simulink model "MDR_AA_TMD_Intercepteur"  (R2019b)
settings: Solver=ode4  StartTime=0.0  StopTime=Inf  FixedStep=0.01  RelTol=1e-3
values from neighbouring files (symbols this model uses):
  stdatm = [0 100 200 300 400 500 600 700 800 900 1000 1100 ... (4305 elements, 861x5)]    [stdatm.mat]
undefined symbols (not defined in the file or in its folder): Aero_Struct_CM, Aero_TMD, e0_0, e1_0, e2_0, e3_0, magnitude, Masse_Inertie_TMD, pow, Propu_TMD, Simu_TMD, Vm_0, xme_0
libraries: simulink x17
(part 3 of 4)

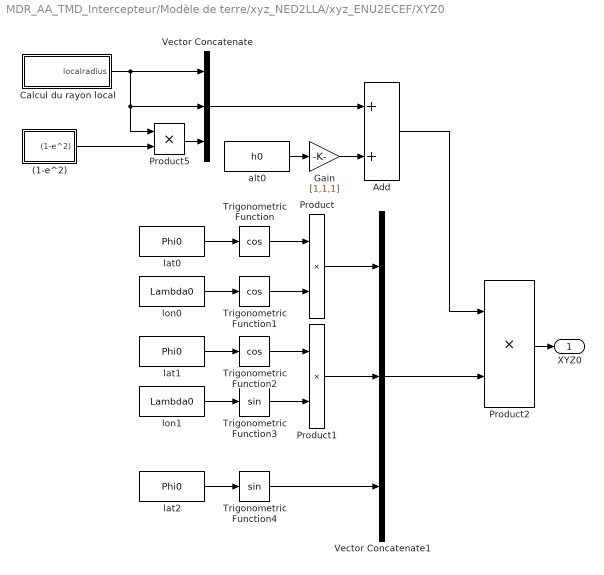
== system MDR_AA_TMD_Intercepteur/Modèle de terre/xyz_NED2LLA/xyz_ENU2ECEF/XYZ0 ==
  (1-e^2) : Subsystem
  Add : Sum
  Calcul du rayon local : Subsystem
  Gain : Gain  Gain=[1,1,1]
  Product{,1..2,5} (4 alike) : Product
  Trigonometric Function : Trigonometry  Operator=cos
  Trigonometric Function1 : Trigonometry  Operator=cos
  Trigonometric Function2 : Trigonometry  Operator=cos
  Trigonometric Function3 : Trigonometry
  Trigonometric Function4 : Trigonometry
  Vector Concatenate : Concatenate  NumInputs=3
  Vector Concatenate1 : Concatenate  NumInputs=3
  alt0 : Constant  Value=h0
  lat0 : Constant  Value=Phi0
  lat1 : Constant  Value=Phi0
  lat2 : Constant  Value=Phi0
  lon0 : Constant  Value=Lambda0
  lon1 : Constant  Value=Lambda0
  XYZ0 : Outport  VectorParamsAs1DForOutWhenUnconnected=off
  wires:
  Calcul du rayon local/1(localradius) -> Product5/1, Vector Concatenate/2, Vector Concatenate/1
  Product2/1 -> XYZ0/1
  Trigonometric Function4/1 -> Vector Concatenate1/3
  Add/1 -> Product2/1
  Product5/1 -> Vector Concatenate/3
  lon1/1 -> Trigonometric Function3/1
  Trigonometric Function2/1 -> Product1/1
  Trigonometric Function3/1 -> Product1/2
  Trigonometric Function1/1 -> Product/2
  Product1/1 -> Vector Concatenate1/2
  Gain/1 -> Add/2
  Trigonometric Function/1 -> Product/1
  lat1/1 -> Trigonometric Function2/1
  Product/1 -> Vector Concatenate1/1
  alt0/1 -> Gain/1
  lon0/1 -> Trigonometric Function1/1
  lat0/1 -> Trigonometric Function/1
  Vector Concatenate/1 -> Add/1
  (1-e^2)/1((1-e^2)) -> Product5/2
  lat2/1 -> Trigonometric Function4/1
  Vector Concatenate1/1 -> Product2/2

== system MDR_AA_TMD_Intercepteur/Cible/Cible Cinématique v1.1/Actionneur Simulight/Retard Angle/Gestion division par 0 ==
  Zero_Possible : Inport
  IC : InitialCondition  Value=0.01
  Memory : Memory
  Switch : Switch  Criteria=u2 ~= 0
  Non_zero : Outport  VectorParamsAs1DForOutWhenUnconnected=off
  wires:
  IC/1 -> Non_zero/1
  Memory/1 -> Switch/3
  Switch/1 -> IC/1, Memory/1
  Zero_Possible/1 -> Switch/2, Switch/1

== system MDR_AA_TMD_Intercepteur/Cible/Cible Cinématique v1.1/Actionneur Simulight1/Retard Angle/Gestion division par 0 ==
  Zero_Possible : Inport
  IC : InitialCondition  Value=0.01
  Memory : Memory
  Switch : Switch  Criteria=u2 ~= 0
  Non_zero : Outport  VectorParamsAs1DForOutWhenUnconnected=off
  wires:
  IC/1 -> Non_zero/1
  Memory/1 -> Switch/3
  Switch/1 -> IC/1, Memory/1
  Zero_Possible/1 -> Switch/2, Switch/1

== system MDR_AA_TMD_Intercepteur/Cible/Cible Cinématique v1.1/Cinématique 6ddl Simulight avec pilotage en force/Calcul de la vitesse engin dans le repère inertiel/Quaternion2DCM ==
  note: Output
  note: Assemble Body-Inertial DCM
  Quaternion : Inport  PortDimensions=[4 1]
  1-2q1^2-2q2^2 : Fcn  Expr=1-2*u(2)^2-2*u(3)^2
  1-2q1^2-2q3^2 : Fcn  Expr=1-2*u(2)^2-2*u(4)^2
  1-2q2^2-2q3^2 : Fcn  Expr=1-2*u(3)^2-2*u(4)^2
  2q1q2+2q0q3 : Fcn  Expr=2*u(2)*u(3)+2*u(1)*u(4)
  2q1q2-2q0q3 : Fcn  Expr=2*u(2)*u(3)-2*u(1)*u(4)
  2q1q3+2q0q2 : Fcn  Expr=2*u(2)*u(4)+2*u(1)*u(3)
  2q1q3-2q0q2 : Fcn  Expr=2*u(2)*u(4)-2*u(1)*u(3)
  2q2q3+2q0q1 : Fcn  Expr=2*u(3)*u(4)+2*u(1)*u(2)
  2q2q3-2q0q1 : Fcn  Expr=2*u(3)*u(4)-2*u(1)*u(2)
  Math Function : Math  Operator=transpose  SaturateOnIntegerOverflow=on
  Rbi Matrix : Concatenate  NumInputs=3  Mode=Multidimensional array  ConcatenateDimension=2
  Rbi Col1 : Concatenate  NumInputs=3  Mode=Multidimensional array
  Rbi Col2 : Concatenate  NumInputs=3  Mode=Multidimensional array
  Rbi Col3 : Concatenate  NumInputs=3  Mode=Multidimensional array
  DCM : Outport  VectorParamsAs1DForOutWhenUnconnected=off
  wires:
  Math Function/1 -> DCM/1
  Rbi Matrix/1 -> Math Function/1
  Rbi Col1/1 -> Rbi Matrix/1
  1-2q2^2-2q3^2/1 -> Rbi Col1/1
  2q1q2+2q0q3/1 -> Rbi Col1/2
  2q1q3-2q0q2/1 -> Rbi Col1/3
  2q1q2-2q0q3/1 -> Rbi Col2/1
  1-2q1^2-2q3^2/1 -> Rbi Col2/2
  2q2q3+2q0q1/1 -> Rbi Col2/3
  2q1q3+2q0q2/1 -> Rbi Col3/1
  2q2q3-2q0q1/1 -> Rbi Col3/2
  1-2q1^2-2q2^2/1 -> Rbi Col3/3
  Rbi Col2/1 -> Rbi Matrix/2
  Rbi Col3/1 -> Rbi Matrix/3
  Quaternion/1 -> 1-2q2^2-2q3^2/1, 2q1q2+2q0q3/1, 2q1q3-2q0q2/1, 2q1q2-2q0q3/1, 2q2q3-2q0q1/1, 1-2q1^2-2q2^2/1, 2q1q3+2q0q2/1, 2q2q3+2q0q1/1, 1-2q1^2-2q3^2/1

== system MDR_AA_TMD_Intercepteur/Cible/Cible Cinématique v1.1/Cinématique 6ddl Simulight avec pilotage en force/Calcul des pqr/pqr_a ==
  AlphaR : Inport
  BetaR : Inport  Port=2
  Constant : Constant  Value=0
  Vector Concatenate : Concatenate  NumInputs=3
  dérive alpha/beta : Subsystem
  pqr_a : Outport  VectorParamsAs1DForOutWhenUnconnected=off
  wires:
  AlphaR/1 -> dérive alpha/beta/1(AlphaR)
  BetaR/1 -> dérive alpha/beta/2(BetaR)
  dérive alpha/beta/2(dBetaR) -> Vector Concatenate/3
  dérive alpha/beta/1(dAlphaR) -> Vector Concatenate/2
  Constant/1 -> Vector Concatenate/1
  Vector Concatenate/1 -> pqr_a/1

== system MDR_AA_TMD_Intercepteur/Cible/Cible Cinématique v1.1/Cinématique 6ddl Simulight avec pilotage en force/Calcul des pqr/pqr_b ==
  Ab : Inport
  Vb : Inport  Port=2
  Divide : Product  Inputs=*/
  Gain : Gain  Gain=[0 -1 1]
  Selector : Selector  InputPortWidth=3  IndexOptions=Index vector (dialog)  Indices=[1]  OutputSizes=1
  Selector1 : Selector  InputPortWidth=3  IndexOptions=Index vector (dialog)  Indices=[1 3 2]  OutputSizes=1
  pqr_b : Outport  VectorParamsAs1DForOutWhenUnconnected=off
  wires:
  Selector/1 -> Divide/2
  Ab/1 -> Selector1/1
  Vb/1 -> Selector/1
  Divide/1 -> Gain/1
  Gain/1 -> pqr_b/1
  Selector1/1 -> Divide/1

== system MDR_AA_TMD_Intercepteur/Cible/Cible Cinématique v1.1/Cinématique 6ddl Simulight avec pilotage en force/Equations des forces/Gestion de sortie de rampe ==
  Fm : Inport
  Compare To Constant : simulink/Logic and Bit Operations/Compare To Constant  relop=>  const=Longueur_Missile/1000  OutDataTypeStr=boolean
  Integrator : Integrator
  Integrator1 : Integrator  InitialCondition=[0 0 0]
  Norme : Subsystem  mask(Norme){}
      mask help: Calcul la norme quadratique d'un vecteur.
      mask Help: eval('OpenHelp(''A3_NG.mdl'', ''Help\html\A3_NG_Model_Norme.html'')');
  Saturation : Saturate  UpperLimit=inf  LowerLimit=0
  Selector1 : Selector  InputPortWidth=3  IndexOptions=Index vector (dialog)  Indices=[1]  OutputSizes=1
  Sortie_Rampe : Outport  VectorParamsAs1DForOutWhenUnconnected=off
  wires:
  Integrator1/1 -> Norme/1(V)
  Norme/1(||V||) -> Compare To Constant/1
  Integrator/1 -> Integrator1/1
  Compare To Constant/1 -> Sortie_Rampe/1
  Selector1/1 -> Saturation/1
  Saturation/1 -> Integrator/1
  Fm/1 -> Selector1/1

== system MDR_AA_TMD_Intercepteur/Cible/Cible Cinématique v1.1/Cinématique 6ddl Simulight avec pilotage en force/Equations des forces/Sous contrainte de la rampe, effort uniquement sur l'axe longitudinal ==
  F : Inport
  Constant : Constant  Value=0
  Constant1 : Constant  Value=0
  Saturation : Saturate  UpperLimit=inf  LowerLimit=0
  Selector1 : Selector  InputPortWidth=3  IndexOptions=Index vector (dialog)  Indices=[1]  OutputSizes=1
  Vector Concatenate : Concatenate  NumInputs=3
  Fx : Outport  VectorParamsAs1DForOutWhenUnconnected=off
  wires:
  F/1 -> Selector1/1
  Selector1/1 -> Saturation/1
  Saturation/1 -> Vector Concatenate/1
  Vector Concatenate/1 -> Fx/1
  Constant/1 -> Vector Concatenate/2
  Constant1/1 -> Vector Concatenate/3

== system MDR_AA_TMD_Intercepteur/Cible/Cible Cinématique v1.1/Cinématique 6ddl Simulight avec pilotage en force/Equations des forces/U^V ==
  a(1) a(2) a(3) : Inport
  b(1) b(2) b(3) : Inport  Port=2
  Product : Product  SaturateOnIntegerOverflow=on  RndMeth=Zero  InputSameDT=on  OutDataTypeStr=Inherit: Same as first input
  Product1 : Product  SaturateOnIntegerOverflow=on  RndMeth=Zero  InputSameDT=on  OutDataTypeStr=Inherit: Same as first input
  Selector : Selector  InputPortWidth=3  IndexOptions=Index vector (dialog)  Indices=[2 3 1]  OutputSizes=1
  Selector1 : Selector  InputPortWidth=3  IndexOptions=Index vector (dialog)  Indices=[3 1 2]  OutputSizes=1
  Selector2 : Selector  InputPortWidth=3  IndexOptions=Index vector (dialog)  Indices=[2 3 1]  OutputSizes=1
  Selector3 : Selector  InputPortWidth=3  IndexOptions=Index vector (dialog)  Indices=[3 1 2]  OutputSizes=1
  Sum : Sum  Inputs=+|-  SaturateOnIntegerOverflow=on  InputSameDT=on  OutDataTypeStr=Inherit: Same as first input
  c(1) c(2) c(3) : Outport  VectorParamsAs1DForOutWhenUnconnected=off
  wires:
  Sum/1 -> c(1) c(2) c(3)/1
  b(1) b(2) b(3)/1 -> Selector1/1, Selector2/1
  Selector/1 -> Product/1
  a(1) a(2) a(3)/1 -> Selector/1, Selector3/1
  Product/1 -> Sum/1
  Selector1/1 -> Product/2
  Product1/1 -> Sum/2
  Selector2/1 -> Product1/2
  Selector3/1 -> Product1/1

== system MDR_AA_TMD_Intercepteur/Cible/Cible Cinématique v1.1/Cinématique 6ddl Simulight avec pilotage en force/Pesanteur/Inert2Miss ==
  Euler : Inport
  U : Inport  Port=2
  Euler2DCM : Subsystem  mask(Euler2DCM){}
      mask help:
      | Calcul la matrice de passage DCM (Direct Cosine Matrix) à partir des angles d'Euler.
      |
      | DCM :=[
      | [c(theta)c(psi)	-c(phi)s(psi)+s(phi)s(theta)c(psi)	s(phi)s(psi)+c(phi)s(theta)c(psi)
      |
      | c(theta)s(psi)	c(phi)c(psi)+s(phi)s(theta)s(psi)	-s(phi)c(psi)+c(phi)s(theta)s(psi)
      |
      | -s(theta)		s(phi)c(theta)			c(phi)c(theta)
      | ]^T
      | où c correspond à cos,  et s correspond à sin
      mask Help: eval('OpenHelp(''A3_NG.mdl'', ''Help\html\A3_NG_Model_Euler2DCM.html'')');
  Product : Product  Multiplication=Matrix(*)  RndMeth=Zero
  V : Outport  VectorParamsAs1DForOutWhenUnconnected=off
  wires:
  Euler2DCM/1(DCM) -> Product/1
  Product/1 -> V/1
  U/1 -> Product/2
  Euler/1 -> Euler2DCM/1(Euler)

== system MDR_AA_TMD_Intercepteur/Cible/Cible Cinématique v1.1/Cinématique 6ddl Simulight avec pilotage en force/pqr2Quaternion/Euler2Quaternion ==
  note: Sources
  note: Attitude trigonometry
  Euler : Inport  PortDimensions=[3 1]
  1/2 : Gain  Gain=1/2  SaturateOnIntegerOverflow=on  OutDataTypeStr=Inherit: Same as input  ParamDataTypeStr=Inherit: Same as input
  Demux : Demux  Outputs=3
  Fcn4 : Fcn  Expr=u(2)*u(4)*u(6)+u(1)*u(3)*u(5)
  Fcn5 : Fcn  Expr=u(1)*u(4)*u(6)-u(2)*u(3)*u(5)
  Fcn6 : Fcn  Expr=u(2)*u(3)*u(6)+u(1)*u(4)*u(5)
  Fcn7 : Fcn  Expr=u(2)*u(4)*u(5)-u(1)*u(3)*u(6)
  Mux1 : Mux  Inputs=6
  Mux3 : Mux
  cos(phi/2) : Trigonometry  Operator=cos
  cos(psi/2) : Trigonometry  Operator=cos
  cos(theta/2) : Trigonometry  Operator=cos
  sin(phi/2) : Trigonometry
  sin(psi/2) : Trigonometry
  sin(theta/2) : Trigonometry
  Quaternion : Outport  VectorParamsAs1DForOutWhenUnconnected=off
  wires:
  Fcn7/1 -> Mux3/4
  Fcn6/1 -> Mux3/3
  Fcn5/1 -> Mux3/2
  Fcn4/1 -> Mux3/1
  Mux3/1 -> Quaternion/1
  Mux1/1 -> Fcn7/1, Fcn6/1, Fcn4/1, Fcn5/1
  cos(psi/2)/1 -> Mux1/6
  sin(psi/2)/1 -> Mux1/5
  cos(theta/2)/1 -> Mux1/4
  sin(theta/2)/1 -> Mux1/3
  cos(phi/2)/1 -> Mux1/2
  sin(phi/2)/1 -> Mux1/1
  Euler/1 -> 1/2/1
  1/2/1 -> Demux/1
  Demux/1 -> sin(phi/2)/1, cos(phi/2)/1
  Demux/2 -> cos(theta/2)/1, sin(theta/2)/1
  Demux/3 -> cos(psi/2)/1, sin(psi/2)/1

== system MDR_AA_TMD_Intercepteur/Cible/Cible Cinématique v1.1/Cinématique 6ddl Simulight avec pilotage en force/pqr2Quaternion/Norme ==
  V : Inport
  Dot Product : DotProduct  InputSameDT=on  OutDataTypeStr=Inherit: Inherit via internal rule
  Sqrt : Math  Operator=sqrt  SaturateOnIntegerOverflow=on
  ||V|| : Outport  VectorParamsAs1DForOutWhenUnconnected=off
  wires:
  Sqrt/1 -> ||V||/1
  V/1 -> Dot Product/2, Dot Product/1
  Dot Product/1 -> Sqrt/1

== system MDR_AA_TMD_Intercepteur/Cible/Cible Cinématique v1.1/Cinématique 6ddl Simulight avec pilotage en force/pqr2Quaternion/pqr to eidot ==
  pqr : Inport
  e0e1e2e3 : Inport  Port=2
  Gain : Gain  Gain=100  SaturateOnIntegerOverflow=on  OutDataTypeStr=Inherit: Same as input  ParamDataTypeStr=Inherit: Same as input
  Mux1 : Mux  Inputs=[3 4 1]
  Mux2 : Mux
  e0dot : Fcn  Expr=-0.5 * ( u[5]*u[1]+u[6]*u[2]+u[7]*u[3] )
  e1dot : Fcn  Expr=0.5 * ( u[4]*u[1]+u[6]*u[3]-u[7]*u[2] )
  e2dot : Fcn  Expr=0.5 * ( u[4]*u[2]+u[7]*u[1]-u[5]*u[3] )
  e3dot : Fcn  Expr=0.5 * ( u[4]*u[3]+u[5]*u[2]-u[6]*u[1] )
  lambda : Fcn  Expr=1-( pow(u[1],2) + pow(u[2],2) + pow(u[3],2) + pow(u[4],2) )
  eidot : Outport  VectorParamsAs1DForOutWhenUnconnected=off
  wires:
  e0e1e2e3/1 -> Mux1/2, lambda/1
  Gain/1 -> Mux1/3
  lambda/1 -> Gain/1
  e3dot/1 -> Mux2/4
  Mux1/1 -> e3dot/1, e2dot/1, e1dot/1, e0dot/1
  e2dot/1 -> Mux2/3
  e1dot/1 -> Mux2/2
  e0dot/1 -> Mux2/1
  pqr/1 -> Mux1/1
  Mux2/1 -> eidot/1

== system MDR_AA_TMD_Intercepteur/Cible/Cible Cinématique v1.1/Pilote 2 axes Simulight à partir de gradient/Alpha commandé - Plan de tangage/Zero Offset ==
  In : Inport
  Abs : Abs  SaturateOnIntegerOverflow=on
  Constant : Constant  Value=tol
  Non-zero Sign : Subsystem  mask(Non-zero sign){}
      mask help: Sign function outputs 1 for input greater than or equal to 0, and -1 otherwise.
  Product : Product  SaturateOnIntegerOverflow=on  RndMeth=Zero  InputSameDT=on  OutDataTypeStr=Inherit: Same as first input
  Switch : Switch  Threshold=tol  SaturateOnIntegerOverflow=on  InputSameDT=on
  Out : Outport  VectorParamsAs1DForOutWhenUnconnected=off
  wires:
  Switch/1 -> Out/1
  Product/1 -> Switch/3
  Constant/1 -> Product/2
  Non-zero Sign/1(Out) -> Product/1
  Abs/1 -> Switch/2
  In/1 -> Abs/1, Non-zero Sign/1(In), Switch/1

== system MDR_AA_TMD_Intercepteur/Cible/Cible Cinématique v1.1/Pilote 2 axes Simulight à partir de gradient/Beta commandé - Plan de lacet/Zero Offset ==
  In : Inport
  Abs : Abs  SaturateOnIntegerOverflow=on
  Constant : Constant  Value=tol
  Non-zero Sign : Subsystem  mask(Non-zero sign){}
      mask help: Sign function outputs 1 for input greater than or equal to 0, and -1 otherwise.
  Product : Product  SaturateOnIntegerOverflow=on  RndMeth=Zero  InputSameDT=on  OutDataTypeStr=Inherit: Same as first input
  Switch : Switch  Threshold=tol  SaturateOnIntegerOverflow=on  InputSameDT=on
  Out : Outport  VectorParamsAs1DForOutWhenUnconnected=off
  wires:
  In/1 -> Switch/1, Non-zero Sign/1(In), Abs/1
  Abs/1 -> Switch/2
  Non-zero Sign/1(Out) -> Product/1
  Constant/1 -> Product/2
  Product/1 -> Switch/3
  Switch/1 -> Out/1

== system MDR_AA_TMD_Intercepteur/Intercepteur_TMD/Auto-Directeur/Autodirecteur Parfait v1.0/Calcul du vecteur rotation instantané de la droite missile//but dans le repère inertiel/Norme ==
  V : Inport
  Dot Product : DotProduct  InputSameDT=on  OutDataTypeStr=Inherit: Inherit via internal rule
  Sqrt : Math  Operator=sqrt  SaturateOnIntegerOverflow=on
  ||V|| : Outport  VectorParamsAs1DForOutWhenUnconnected=off
  wires:
  Sqrt/1 -> ||V||/1
  V/1 -> Dot Product/2, Dot Product/1
  Dot Product/1 -> Sqrt/1

== system MDR_AA_TMD_Intercepteur/Intercepteur_TMD/Auto-Directeur/Autodirecteur Parfait v1.0/Calcul du vecteur rotation instantané de la droite missile//but dans le repère inertiel/U^V ==
  a(1) a(2) a(3) : Inport
  b(1) b(2) b(3) : Inport  Port=2
  Product : Product  SaturateOnIntegerOverflow=on  RndMeth=Zero  InputSameDT=on  OutDataTypeStr=Inherit: Same as first input
  Product1 : Product  SaturateOnIntegerOverflow=on  RndMeth=Zero  InputSameDT=on  OutDataTypeStr=Inherit: Same as first input
  Selector : Selector  InputPortWidth=3  IndexOptions=Index vector (dialog)  Indices=[2 3 1]  OutputSizes=1
  Selector1 : Selector  InputPortWidth=3  IndexOptions=Index vector (dialog)  Indices=[3 1 2]  OutputSizes=1
  Selector2 : Selector  InputPortWidth=3  IndexOptions=Index vector (dialog)  Indices=[2 3 1]  OutputSizes=1
  Selector3 : Selector  InputPortWidth=3  IndexOptions=Index vector (dialog)  Indices=[3 1 2]  OutputSizes=1
  Sum : Sum  Inputs=+|-  SaturateOnIntegerOverflow=on  InputSameDT=on  OutDataTypeStr=Inherit: Same as first input
  c(1) c(2) c(3) : Outport  VectorParamsAs1DForOutWhenUnconnected=off
  wires:
  Sum/1 -> c(1) c(2) c(3)/1
  b(1) b(2) b(3)/1 -> Selector1/1, Selector2/1
  Selector/1 -> Product/1
  a(1) a(2) a(3)/1 -> Selector/1, Selector3/1
  Product/1 -> Sum/1
  Selector1/1 -> Product/2
  Product1/1 -> Sum/2
  Selector2/1 -> Product1/2
  Selector3/1 -> Product1/1

== system MDR_AA_TMD_Intercepteur/Intercepteur_TMD/Auto-Directeur/Autodirecteur Parfait v1.0/Changement de repère inertiel -> miss/Inert2Miss1 ==
  Euler : Inport
  U : Inport  Port=2
  Euler2DCM : Subsystem  mask(Euler2DCM){}
      mask help:
      | Calcul la matrice de passage DCM (Direct Cosine Matrix) à partir des angles d'Euler.
      |
      | DCM :=[
      | [c(theta)c(psi)	-c(phi)s(psi)+s(phi)s(theta)c(psi)	s(phi)s(psi)+c(phi)s(theta)c(psi)
      |
      | c(theta)s(psi)	c(phi)c(psi)+s(phi)s(theta)s(psi)	-s(phi)c(psi)+c(phi)s(theta)s(psi)
      |
      | -s(theta)		s(phi)c(theta)			c(phi)c(theta)
      | ]^T
      | où c correspond à cos,  et s correspond à sin
      mask Help: eval('OpenHelp(''A3_NG.mdl'', ''Help\html\A3_NG_Model_Euler2DCM.html'')');
  Product : Product  Multiplication=Matrix(*)  RndMeth=Zero
  V : Outport  VectorParamsAs1DForOutWhenUnconnected=off
  wires:
  Euler2DCM/1(DCM) -> Product/1
  Product/1 -> V/1
  U/1 -> Product/2
  Euler/1 -> Euler2DCM/1(Euler)

== system MDR_AA_TMD_Intercepteur/Intercepteur_TMD/Auto-Directeur/Autodirecteur Parfait v1.0/Site et Gisement de la droite missile//but dans le repère inertiel/Norme ==
  V : Inport
  Dot Product : DotProduct  InputSameDT=on  OutDataTypeStr=Inherit: Inherit via internal rule
  Sqrt : Math  Operator=sqrt  SaturateOnIntegerOverflow=on
  ||V|| : Outport  VectorParamsAs1DForOutWhenUnconnected=off
  wires:
  Sqrt/1 -> ||V||/1
  V/1 -> Dot Product/2, Dot Product/1
  Dot Product/1 -> Sqrt/1

== system MDR_AA_TMD_Intercepteur/Intercepteur_TMD/Bloc Cinématique/Cinématique 6ddl Simulight avec pilotage en force/Calcul de la vitesse engin dans le repère inertiel/Quaternion2DCM ==
  note: Output
  note: Assemble Body-Inertial DCM
  Quaternion : Inport  PortDimensions=[4 1]
  1-2q1^2-2q2^2 : Fcn  Expr=1-2*u(2)^2-2*u(3)^2
  1-2q1^2-2q3^2 : Fcn  Expr=1-2*u(2)^2-2*u(4)^2
  1-2q2^2-2q3^2 : Fcn  Expr=1-2*u(3)^2-2*u(4)^2
  2q1q2+2q0q3 : Fcn  Expr=2*u(2)*u(3)+2*u(1)*u(4)
  2q1q2-2q0q3 : Fcn  Expr=2*u(2)*u(3)-2*u(1)*u(4)
  2q1q3+2q0q2 : Fcn  Expr=2*u(2)*u(4)+2*u(1)*u(3)
  2q1q3-2q0q2 : Fcn  Expr=2*u(2)*u(4)-2*u(1)*u(3)
  2q2q3+2q0q1 : Fcn  Expr=2*u(3)*u(4)+2*u(1)*u(2)
  2q2q3-2q0q1 : Fcn  Expr=2*u(3)*u(4)-2*u(1)*u(2)
  Math Function : Math  Operator=transpose  SaturateOnIntegerOverflow=on
  Rbi Matrix : Concatenate  NumInputs=3  Mode=Multidimensional array  ConcatenateDimension=2
  Rbi Col1 : Concatenate  NumInputs=3  Mode=Multidimensional array
  Rbi Col2 : Concatenate  NumInputs=3  Mode=Multidimensional array
  Rbi Col3 : Concatenate  NumInputs=3  Mode=Multidimensional array
  DCM : Outport  VectorParamsAs1DForOutWhenUnconnected=off
  wires:
  Math Function/1 -> DCM/1
  Rbi Matrix/1 -> Math Function/1
  Rbi Col1/1 -> Rbi Matrix/1
  1-2q2^2-2q3^2/1 -> Rbi Col1/1
  2q1q2+2q0q3/1 -> Rbi Col1/2
  2q1q3-2q0q2/1 -> Rbi Col1/3
  2q1q2-2q0q3/1 -> Rbi Col2/1
  1-2q1^2-2q3^2/1 -> Rbi Col2/2
  2q2q3+2q0q1/1 -> Rbi Col2/3
  2q1q3+2q0q2/1 -> Rbi Col3/1
  2q2q3-2q0q1/1 -> Rbi Col3/2
  1-2q1^2-2q2^2/1 -> Rbi Col3/3
  Rbi Col2/1 -> Rbi Matrix/2
  Rbi Col3/1 -> Rbi Matrix/3
  Quaternion/1 -> 1-2q2^2-2q3^2/1, 2q1q2+2q0q3/1, 2q1q3-2q0q2/1, 2q1q2-2q0q3/1, 2q2q3-2q0q1/1, 1-2q1^2-2q2^2/1, 2q1q3+2q0q2/1, 2q2q3+2q0q1/1, 1-2q1^2-2q3^2/1

== system MDR_AA_TMD_Intercepteur/Intercepteur_TMD/Bloc Cinématique/Cinématique 6ddl Simulight avec pilotage en force/Calcul des pqr/pqr_a ==
  AlphaR : Inport
  BetaR : Inport  Port=2
  Constant : Constant  Value=0
  Vector Concatenate : Concatenate  NumInputs=3
  dérive alpha/beta : Subsystem
  pqr_a : Outport  VectorParamsAs1DForOutWhenUnconnected=off
  wires:
  AlphaR/1 -> dérive alpha/beta/1(AlphaR)
  BetaR/1 -> dérive alpha/beta/2(BetaR)
  dérive alpha/beta/2(dBetaR) -> Vector Concatenate/3
  dérive alpha/beta/1(dAlphaR) -> Vector Concatenate/2
  Constant/1 -> Vector Concatenate/1
  Vector Concatenate/1 -> pqr_a/1

== system MDR_AA_TMD_Intercepteur/Intercepteur_TMD/Bloc Cinématique/Cinématique 6ddl Simulight avec pilotage en force/Calcul des pqr/pqr_b ==
  Ab : Inport
  Vb : Inport  Port=2
  Divide : Product  Inputs=*/
  Gain : Gain  Gain=[0 -1 1]
  Selector : Selector  InputPortWidth=3  IndexOptions=Index vector (dialog)  Indices=[1]  OutputSizes=1
  Selector1 : Selector  InputPortWidth=3  IndexOptions=Index vector (dialog)  Indices=[1 3 2]  OutputSizes=1
  pqr_b : Outport  VectorParamsAs1DForOutWhenUnconnected=off
  wires:
  Selector/1 -> Divide/2
  Ab/1 -> Selector1/1
  Vb/1 -> Selector/1
  Divide/1 -> Gain/1
  Gain/1 -> pqr_b/1
  Selector1/1 -> Divide/1

== system MDR_AA_TMD_Intercepteur/Intercepteur_TMD/Bloc Cinématique/Cinématique 6ddl Simulight avec pilotage en force/Equations des forces/Gestion de sortie de rampe ==
  Fm : Inport
  Compare To Constant : simulink/Logic and Bit Operations/Compare To Constant  relop=>  const=Longueur_Missile/1000  OutDataTypeStr=boolean
  Integrator : Integrator
  Integrator1 : Integrator  InitialCondition=[0 0 0]
  Norme : Subsystem  mask(Norme){}
      mask help: Calcul la norme quadratique d'un vecteur.
      mask Help: eval('OpenHelp(''A3_NG.mdl'', ''Help\html\A3_NG_Model_Norme.html'')');
  Saturation : Saturate  UpperLimit=inf  LowerLimit=0
  Selector1 : Selector  InputPortWidth=3  IndexOptions=Index vector (dialog)  Indices=[1]  OutputSizes=1
  Sortie_Rampe : Outport  VectorParamsAs1DForOutWhenUnconnected=off
  wires:
  Integrator1/1 -> Norme/1(V)
  Norme/1(||V||) -> Compare To Constant/1
  Integrator/1 -> Integrator1/1
  Compare To Constant/1 -> Sortie_Rampe/1
  Selector1/1 -> Saturation/1
  Saturation/1 -> Integrator/1
  Fm/1 -> Selector1/1

== system MDR_AA_TMD_Intercepteur/Intercepteur_TMD/Bloc Cinématique/Cinématique 6ddl Simulight avec pilotage en force/Equations des forces/Sous contrainte de la rampe, effort uniquement sur l'axe longitudinal ==
  F : Inport
  Constant : Constant  Value=0
  Constant1 : Constant  Value=0
  Saturation : Saturate  UpperLimit=inf  LowerLimit=0
  Selector1 : Selector  InputPortWidth=3  IndexOptions=Index vector (dialog)  Indices=[1]  OutputSizes=1
  Vector Concatenate : Concatenate  NumInputs=3
  Fx : Outport  VectorParamsAs1DForOutWhenUnconnected=off
  wires:
  F/1 -> Selector1/1
  Selector1/1 -> Saturation/1
  Saturation/1 -> Vector Concatenate/1
  Vector Concatenate/1 -> Fx/1
  Constant/1 -> Vector Concatenate/2
  Constant1/1 -> Vector Concatenate/3

== system MDR_AA_TMD_Intercepteur/Intercepteur_TMD/Bloc Cinématique/Cinématique 6ddl Simulight avec pilotage en force/Equations des forces/U^V ==
  a(1) a(2) a(3) : Inport
  b(1) b(2) b(3) : Inport  Port=2
  Product : Product  SaturateOnIntegerOverflow=on  RndMeth=Zero  InputSameDT=on  OutDataTypeStr=Inherit: Same as first input
  Product1 : Product  SaturateOnIntegerOverflow=on  RndMeth=Zero  InputSameDT=on  OutDataTypeStr=Inherit: Same as first input
  Selector : Selector  InputPortWidth=3  IndexOptions=Index vector (dialog)  Indices=[2 3 1]  OutputSizes=1
  Selector1 : Selector  InputPortWidth=3  IndexOptions=Index vector (dialog)  Indices=[3 1 2]  OutputSizes=1
  Selector2 : Selector  InputPortWidth=3  IndexOptions=Index vector (dialog)  Indices=[2 3 1]  OutputSizes=1
  Selector3 : Selector  InputPortWidth=3  IndexOptions=Index vector (dialog)  Indices=[3 1 2]  OutputSizes=1
  Sum : Sum  Inputs=+|-  SaturateOnIntegerOverflow=on  InputSameDT=on  OutDataTypeStr=Inherit: Same as first input
  c(1) c(2) c(3) : Outport  VectorParamsAs1DForOutWhenUnconnected=off
  wires:
  Sum/1 -> c(1) c(2) c(3)/1
  b(1) b(2) b(3)/1 -> Selector1/1, Selector2/1
  Selector/1 -> Product/1
  a(1) a(2) a(3)/1 -> Selector/1, Selector3/1
  Product/1 -> Sum/1
  Selector1/1 -> Product/2
  Product1/1 -> Sum/2
  Selector2/1 -> Product1/2
  Selector3/1 -> Product1/1

== system MDR_AA_TMD_Intercepteur/Intercepteur_TMD/Bloc Cinématique/Cinématique 6ddl Simulight avec pilotage en force/Pesanteur/Inert2Miss ==
  Euler : Inport
  U : Inport  Port=2
  Euler2DCM : Subsystem  mask(Euler2DCM){}
      mask help:
      | Calcul la matrice de passage DCM (Direct Cosine Matrix) à partir des angles d'Euler.
      |
      | DCM :=[
      | [c(theta)c(psi)	-c(phi)s(psi)+s(phi)s(theta)c(psi)	s(phi)s(psi)+c(phi)s(theta)c(psi)
      |
      | c(theta)s(psi)	c(phi)c(psi)+s(phi)s(theta)s(psi)	-s(phi)c(psi)+c(phi)s(theta)s(psi)
      |
      | -s(theta)		s(phi)c(theta)			c(phi)c(theta)
      | ]^T
      | où c correspond à cos,  et s correspond à sin
      mask Help: eval('OpenHelp(''A3_NG.mdl'', ''Help\html\A3_NG_Model_Euler2DCM.html'')');
  Product : Product  Multiplication=Matrix(*)  RndMeth=Zero
  V : Outport  VectorParamsAs1DForOutWhenUnconnected=off
  wires:
  Euler2DCM/1(DCM) -> Product/1
  Product/1 -> V/1
  U/1 -> Product/2
  Euler/1 -> Euler2DCM/1(Euler)

== system MDR_AA_TMD_Intercepteur/Intercepteur_TMD/Bloc Cinématique/Cinématique 6ddl Simulight avec pilotage en force/pqr2Quaternion/Euler2Quaternion ==
  note: Sources
  note: Attitude trigonometry
  Euler : Inport  PortDimensions=[3 1]
  1/2 : Gain  Gain=1/2  SaturateOnIntegerOverflow=on  OutDataTypeStr=Inherit: Same as input  ParamDataTypeStr=Inherit: Same as input
  Demux : Demux  Outputs=3
  Fcn4 : Fcn  Expr=u(2)*u(4)*u(6)+u(1)*u(3)*u(5)
  Fcn5 : Fcn  Expr=u(1)*u(4)*u(6)-u(2)*u(3)*u(5)
  Fcn6 : Fcn  Expr=u(2)*u(3)*u(6)+u(1)*u(4)*u(5)
  Fcn7 : Fcn  Expr=u(2)*u(4)*u(5)-u(1)*u(3)*u(6)
  Mux1 : Mux  Inputs=6
  Mux3 : Mux
  cos(phi/2) : Trigonometry  Operator=cos
  cos(psi/2) : Trigonometry  Operator=cos
  cos(theta/2) : Trigonometry  Operator=cos
  sin(phi/2) : Trigonometry
  sin(psi/2) : Trigonometry
  sin(theta/2) : Trigonometry
  Quaternion : Outport  VectorParamsAs1DForOutWhenUnconnected=off
  wires:
  Fcn7/1 -> Mux3/4
  Fcn6/1 -> Mux3/3
  Fcn5/1 -> Mux3/2
  Fcn4/1 -> Mux3/1
  Mux3/1 -> Quaternion/1
  Mux1/1 -> Fcn7/1, Fcn6/1, Fcn4/1, Fcn5/1
  cos(psi/2)/1 -> Mux1/6
  sin(psi/2)/1 -> Mux1/5
  cos(theta/2)/1 -> Mux1/4
  sin(theta/2)/1 -> Mux1/3
  cos(phi/2)/1 -> Mux1/2
  sin(phi/2)/1 -> Mux1/1
  Euler/1 -> 1/2/1
  1/2/1 -> Demux/1
  Demux/1 -> sin(phi/2)/1, cos(phi/2)/1
  Demux/2 -> cos(theta/2)/1, sin(theta/2)/1
  Demux/3 -> cos(psi/2)/1, sin(psi/2)/1

== system MDR_AA_TMD_Intercepteur/Intercepteur_TMD/Bloc Cinématique/Cinématique 6ddl Simulight avec pilotage en force/pqr2Quaternion/Norme ==
  V : Inport
  Dot Product : DotProduct  InputSameDT=on  OutDataTypeStr=Inherit: Inherit via internal rule
  Sqrt : Math  Operator=sqrt  SaturateOnIntegerOverflow=on
  ||V|| : Outport  VectorParamsAs1DForOutWhenUnconnected=off
  wires:
  Sqrt/1 -> ||V||/1
  V/1 -> Dot Product/2, Dot Product/1
  Dot Product/1 -> Sqrt/1

== system MDR_AA_TMD_Intercepteur/Intercepteur_TMD/Bloc Cinématique/Cinématique 6ddl Simulight avec pilotage en force/pqr2Quaternion/pqr to eidot ==
  pqr : Inport
  e0e1e2e3 : Inport  Port=2
  Gain : Gain  Gain=100  SaturateOnIntegerOverflow=on  OutDataTypeStr=Inherit: Same as input  ParamDataTypeStr=Inherit: Same as input
  Mux1 : Mux  Inputs=[3 4 1]
  Mux2 : Mux
  e0dot : Fcn  Expr=-0.5 * ( u[5]*u[1]+u[6]*u[2]+u[7]*u[3] )
  e1dot : Fcn  Expr=0.5 * ( u[4]*u[1]+u[6]*u[3]-u[7]*u[2] )
  e2dot : Fcn  Expr=0.5 * ( u[4]*u[2]+u[7]*u[1]-u[5]*u[3] )
  e3dot : Fcn  Expr=0.5 * ( u[4]*u[3]+u[5]*u[2]-u[6]*u[1] )
  lambda : Fcn  Expr=1-( pow(u[1],2) + pow(u[2],2) + pow(u[3],2) + pow(u[4],2) )
  eidot : Outport  VectorParamsAs1DForOutWhenUnconnected=off
  wires:
  e0e1e2e3/1 -> Mux1/2, lambda/1
  Gain/1 -> Mux1/3
  lambda/1 -> Gain/1
  e3dot/1 -> Mux2/4
  Mux1/1 -> e3dot/1, e2dot/1, e1dot/1, e0dot/1
  e2dot/1 -> Mux2/3
  e1dot/1 -> Mux2/2
  e0dot/1 -> Mux2/1
  pqr/1 -> Mux1/1
  Mux2/1 -> eidot/1

== system MDR_AA_TMD_Intercepteur/Intercepteur_TMD/Calculateur/Guidage/Guidage en Naviguation Proportionnelle 2 axes/Norme ==
  V : Inport
  Dot Product : DotProduct  InputSameDT=on  OutDataTypeStr=Inherit: Inherit via internal rule
  Sqrt : Math  Operator=sqrt  SaturateOnIntegerOverflow=on
  ||V|| : Outport  VectorParamsAs1DForOutWhenUnconnected=off
  wires:
  Sqrt/1 -> ||V||/1
  V/1 -> Dot Product/2, Dot Product/1
  Dot Product/1 -> Sqrt/1

== system MDR_AA_TMD_Intercepteur/Intercepteur_TMD/Calculateur/Pilotage/Pilote 2 axes Simulight avec prise en compte de la manoeuvrabilité max/Alpha commandé - Plan de tangage ==
  GcoV : Inport
  Masse : Inport  Port=2
  Mach : Inport  Port=3
  Pression_dynamique : Inport  Port=4
  Calcul de CN0 : Subsystem
  Calcul du coefficient de CN commandé avec gestion de la division par 0 : Subsystem
  Constant : Constant  Value=vAlpha
  Interpolation linéaire pour trouver l'incidence correspondant au coefficient de portance commandé : Subsystem
  Mach1 : InportShadow  Port=3
  Saturation de CN_co par la valeur max de CN équilibré : Subsystem
  Alphaco : Outport  PortDimensions=1  VectorParamsAs1DForOutWhenUnconnected=off
  wires:
  Calcul du coefficient de CN commandé avec gestion de la division par 0/1(CN_co) -> Saturation de CN_co par la valeur max de CN équilibré/2(CN_co)
  Pression_dynamique/1 -> Calcul du coefficient de CN commandé avec gestion de la division par 0/3(Pression_dynamique)
  Masse/1 -> Calcul du coefficient de CN commandé avec gestion de la division par 0/2(Masse)
  GcoV/1 -> Calcul du coefficient de CN commandé avec gestion de la division par 0/1(GcoV)
  Saturation de CN_co par la valeur max de CN équilibré/1(CN_co_sat) -> Interpolation linéaire pour trouver l'incidence correspondant au coefficient de portance commandé/1(CN_co_sat)
  Mach1/1 -> Saturation de CN_co par la valeur max de CN équilibré/1(Mach)
  Interpolation linéaire pour trouver l'incidence correspondant au coefficient de portance commandé/1(Alphaco) -> Alphaco/1
  Constant/1 -> Interpolation linéaire pour trouver l'incidence correspondant au coefficient de portance commandé/3(vAlpha), Calcul de CN0/1(Alpha)
  Mach/1 -> Calcul de CN0/2(Mach)
  Calcul de CN0/1(vCN0) -> Interpolation linéaire pour trouver l'incidence correspondant au coefficient de portance commandé/2(vCN0)

== system MDR_AA_TMD_Intercepteur/Intercepteur_TMD/Calculateur/Pilotage/Pilote 2 axes Simulight avec prise en compte de la manoeuvrabilité max/Beta commandé - Plan de lacet ==
  GcoH : Inport
  Masse : Inport  Port=2
  Mach : Inport  Port=3
  Pression_dynamique : Inport  Port=4
  Calcul de CY0 : Subsystem
  Calcul du coefficient de CY commandé avec gestion de la division par 0 : Subsystem
  Constant : Constant  Value=vBeta
  Interpolation linéaire pour trouver le dérapage correspondant au coefficient de portance commandé : Subsystem
  Mach1 : InportShadow  Port=3
  Saturation de CN_co par la valeur max de CN équilibré : Subsystem
  Betaco : Outport  PortDimensions=1  VectorParamsAs1DForOutWhenUnconnected=off
  wires:
  Interpolation linéaire pour trouver le dérapage correspondant au coefficient de portance commandé/1(Betaco) -> Betaco/1
  Saturation de CN_co par la valeur max de CN équilibré/1(CY_co_sat) -> Interpolation linéaire pour trouver le dérapage correspondant au coefficient de portance commandé/1(CY_co_sat)
  Calcul de CY0/1(vCY0) -> Interpolation linéaire pour trouver le dérapage correspondant au coefficient de portance commandé/2(vCY0)
  Constant/1 -> Interpolation linéaire pour trouver le dérapage correspondant au coefficient de portance commandé/3(vBeta), Calcul de CY0/1(Beta)
  Mach1/1 -> Saturation de CN_co par la valeur max de CN équilibré/1(Mach)
  Calcul du coefficient de CY commandé avec gestion de la division par 0/1(CY_co) -> Saturation de CN_co par la valeur max de CN équilibré/2(CY_co)
  GcoH/1 -> Calcul du coefficient de CY commandé avec gestion de la division par 0/1(GcoH)
  Masse/1 -> Calcul du coefficient de CY commandé avec gestion de la division par 0/2(Masse)
  Pression_dynamique/1 -> Calcul du coefficient de CY commandé avec gestion de la division par 0/3(Pression_dynamique)
  Mach/1 -> Calcul de CY0/2(Mach)

== system MDR_AA_TMD_Intercepteur/Intercepteur_TMD/Calculateur/Pilotage/Pilote 2 axes Simulight avec prise en compte de la manoeuvrabilité max/Calcul du Mach ==
  Vitesse_Son : Inport
  Vm : Inport  Port=2
  Divide : Product  Inputs=*/
  Norme : Subsystem  mask(Norme){}
      mask help: Calcul la norme quadratique d'un vecteur.
      mask Help: eval('OpenHelp(''A3_NG.mdl'', ''Help\html\A3_NG_Model_Norme.html'')');
  Mach : Outport  VectorParamsAs1DForOutWhenUnconnected=off
  ||V|| : Outport  Port=2  VectorParamsAs1DForOutWhenUnconnected=off
  wires:
  Norme/1(||V||) -> Divide/1, ||V||/1
  Vm/1 -> Norme/1(V)
  Divide/1 -> Mach/1
  Vitesse_Son/1 -> Divide/2

== system MDR_AA_TMD_Intercepteur/Intercepteur_TMD/Calculateur/Pilotage/Pilote 2 axes Simulight avec prise en compte de la manoeuvrabilité max/q\ ==
  ||V|| : Inport
  Rho : Inport  Port=2
  Gain : Gain  Gain=0.5
  Gain1 : Gain  Gain=(Lref^2*pi)/4
  Math Function : Math  Operator=magnitude^2  SaturateOnIntegerOverflow=on
  Product2 : Product  RndMeth=Zero
  rsv2 : Outport  VectorParamsAs1DForOutWhenUnconnected=off
  wires:
  Gain1/1 -> rsv2/1
  Math Function/1 -> Product2/2
  Product2/1 -> Gain1/1
  Rho/1 -> Gain/1
  ||V||/1 -> Math Function/1
  Gain/1 -> Product2/1

== system MDR_AA_TMD_Intercepteur/Intercepteur_TMD/Forces-Moments/Aerodynamique 3D (CA//CY//CN) v1.0/Plan de lacet/Calcul de CN0 ==
  Mach : Inport
  Beta : Inport  Port=2
  CY_0 : Lookup_n-D  BreakpointsForDimension1=vBeta  BreakpointsForDimension2=vMach  BreakpointsForDimension3=Aero_Struct_CM.vBrq  Table=CY  ExtrapMethod=Clip  UseLastTableValue=on  RndMeth=Simplest  InputSameDT=on
  CY0 : Outport  VectorParamsAs1DForOutWhenUnconnected=off
  wires:
  CY_0/1 -> CY0/1
  Mach/1 -> CY_0/2
  Beta/1 -> CY_0/1

== system MDR_AA_TMD_Intercepteur/Intercepteur_TMD/Forces-Moments/Aerodynamique 3D (CA//CY//CN) v1.0/Plan de tangage/Calcul de CN0 ==
  Mach : Inport
  Alpha : Inport  Port=2
  CN_0 : Lookup_n-D  BreakpointsForDimension1=vAlpha  BreakpointsForDimension2=vMach  BreakpointsForDimension3=Aero_Struct_CM.vBrq  Table=CN  ExtrapMethod=Clip  UseLastTableValue=on  RndMeth=Simplest  InputSameDT=on
  CN0 : Outport  VectorParamsAs1DForOutWhenUnconnected=off
  wires:
  Alpha/1 -> CN_0/1
  Mach/1 -> CN_0/2
  CN_0/1 -> CN0/1

== system MDR_AA_TMD_Intercepteur/Intercepteur_TMD/Forces-Moments/Aerodynamique 3D (CA//CY//CN) v1.0/Pression Dynamique Mach/Norme ==
  V : Inport
  Dot Product : DotProduct  InputSameDT=on  OutDataTypeStr=Inherit: Inherit via internal rule
  Sqrt : Math  Operator=sqrt  SaturateOnIntegerOverflow=on
  ||V|| : Outport  VectorParamsAs1DForOutWhenUnconnected=off
  wires:
  Sqrt/1 -> ||V||/1
  V/1 -> Dot Product/2, Dot Product/1
  Dot Product/1 -> Sqrt/1

== system MDR_AA_TMD_Intercepteur/Intercepteur_TMD/Forces-Moments/Aerodynamique 3D (CA//CY//CN) v1.0/Pression Dynamique Mach/q\ ==
  Rho : Inport
  ||V|| : Inport  Port=2
  Gain : Gain  Gain=0.5
  Gain1 : Gain  Gain=(Lref^2*pi)/4
  Math Function : Math  Operator=magnitude^2  SaturateOnIntegerOverflow=on
  Product2 : Product  RndMeth=Zero
  rsv2 : Outport  VectorParamsAs1DForOutWhenUnconnected=off
  wires:
  Gain1/1 -> rsv2/1
  Math Function/1 -> Product2/2
  Product2/1 -> Gain1/1
  Rho/1 -> Gain/1
  ||V||/1 -> Math Function/1
  Gain/1 -> Product2/1

== system MDR_AA_TMD_Intercepteur/Intercepteur_TMD/Forces-Moments/Aerodynamique 3D (CA//CY//CN) v1.0/Trainée/Calcul de CA non propu ==
  Mach : Inport
  Altitude : Inport  Port=2
  CA_ : Lookup_n-D  BreakpointsForDimension1=vAlt  BreakpointsForDimension2=vMach  BreakpointsForDimension3=[0 5 10 15]  Table=CA_np  ExtrapMethod=Clip  UseLastTableValue=on  RndMeth=Simplest  InputSameDT=on
  CA : Outport  VectorParamsAs1DForOutWhenUnconnected=off
  wires:
  CA_/1 -> CA/1
  Mach/1 -> CA_/2
  Altitude/1 -> CA_/1

== system MDR_AA_TMD_Intercepteur/Intercepteur_TMD/Forces-Moments/Aerodynamique 3D (CA//CY//CN) v1.0/Trainée/Calcul de CA propu ==
  Mach : Inport
  Altitude : Inport  Port=2
  CA_ : Lookup_n-D  BreakpointsForDimension1=vAlt  BreakpointsForDimension2=vMach  BreakpointsForDimension3=[0 5 10 15]  Table=CA_p  ExtrapMethod=Clip  UseLastTableValue=on  RndMeth=Simplest  InputSameDT=on
  CA : Outport  VectorParamsAs1DForOutWhenUnconnected=off
  wires:
  CA_/1 -> CA/1
  Mach/1 -> CA_/2
  Altitude/1 -> CA_/1

== system MDR_AA_TMD_Intercepteur/Intercepteur_TMD/Forces-Moments/Propulsion de l'exemple TMD/Propulsion Booster/Calcul de la force de poussée ==
  debit_propu : Inport
  g0 : Inport  Port=2
  Pression_statique : Inport  Port=3
  Calcul de la force de poussée : Subsystem  TreatAsAtomicUnit=on
  If : If  IfExpression=u1 == 0
  Merge : Merge
  Sans force de poussee : Subsystem  TreatAsAtomicUnit=on
  Force_poussee : Outport  VectorParamsAs1DForOutWhenUnconnected=off
  wires:
  debit_propu/1 -> Calcul de la force de poussée/1(debit_propu), If/1
  If/1 -> Sans force de poussee/Action
  If/2 -> Calcul de la force de poussée/Action
  Sans force de poussee/1(Force_poussee) -> Merge/1
  Calcul de la force de poussée/1(Force_poussee) -> Merge/2
  Merge/1 -> Force_poussee/1
  g0/1 -> Calcul de la force de poussée/2(g)
  Pression_statique/1 -> Calcul de la force de poussée/3(Pression_statique)

== system MDR_AA_TMD_Intercepteur/Intercepteur_TMD/Forces-Moments/Propulsion de l'exemple TMD/Propulsion Booster/Calcul du débit de carburant ==
  note: ( 1+ (Rapport_{profil}-1) * (t / t_b) )
  note: ( (Mcombu_{Booster} / t_b) * ( 2 / (1 + Rapport_{Profil}) ) )
  t : Inport
  Add : Sum
  Constant : Constant
  Gain : Gain  Gain=1/t_b
  Gain1 : Gain  Gain=(Booster_Rapport-1)
  Gain3 : Gain  Gain=2/(1+Booster_Rapport)
  Masse combustible / Durée de la phase : Gain  Gain=Booster_Masse/t_b
  debit_propu : Outport  VectorParamsAs1DForOutWhenUnconnected=off
  wires:
  Masse combustible / Durée de la phase/1 -> debit_propu/1
  t/1 -> Gain/1
  Gain/1 -> Gain1/1
  Gain3/1 -> Masse combustible / Durée de la phase/1
  Gain1/1 -> Add/1
  Constant/1 -> Add/2
  Add/1 -> Gain3/1

== system MDR_AA_TMD_Intercepteur/Intercepteur_TMD/Forces-Moments/Propulsion de l'exemple TMD/Propulsion Croisiere/Calcul de la force de poussée ==
  debit_propu : Inport
  g0 : Inport  Port=2
  Pression_statique : Inport  Port=3
  Calcul de la force de poussée : Subsystem  TreatAsAtomicUnit=on
  If : If  IfExpression=u1 == 0
  Merge : Merge
  Sans force de poussee : Subsystem  TreatAsAtomicUnit=on
  Force_poussee : Outport  VectorParamsAs1DForOutWhenUnconnected=off
  wires:
  debit_propu/1 -> Calcul de la force de poussée/1(debit_propu), If/1
  If/1 -> Sans force de poussee/Action
  If/2 -> Calcul de la force de poussée/Action
  Sans force de poussee/1(Force_poussee) -> Merge/1
  Calcul de la force de poussée/1(Force_poussee) -> Merge/2
  Merge/1 -> Force_poussee/1
  g0/1 -> Calcul de la force de poussée/2(g)
  Pression_statique/1 -> Calcul de la force de poussée/3(Pression_statique)

== system MDR_AA_TMD_Intercepteur/Intercepteur_TMD/Forces-Moments/Propulsion de l'exemple TMD/Propulsion Croisiere/Calcul du débit de carburant ==
  note: ( 1+ (Rapport_{profil}-1) * (t / t_b) )
  note: ( (Mcombu_{Booster} / t_b) * ( 2 / (1 + Rapport_{Profil}) ) )
  t : Inport
  Add : Sum
  Constant : Constant
  Gain : Gain  Gain=1/t_b
  Gain1 : Gain  Gain=(Booster_Rapport-1)
  Gain3 : Gain  Gain=2/(1+Booster_Rapport)
  Masse combustible / Durée de la phase : Gain  Gain=Booster_Masse/t_b
  debit_propu : Outport  VectorParamsAs1DForOutWhenUnconnected=off
  wires:
  Masse combustible / Durée de la phase/1 -> debit_propu/1
  t/1 -> Gain/1
  Gain/1 -> Gain1/1
  Gain3/1 -> Masse combustible / Durée de la phase/1
  Gain1/1 -> Add/1
  Constant/1 -> Add/2
  Add/1 -> Gain3/1

== system MDR_AA_TMD_Intercepteur/Modèle de terre/xyz_NED2LLA/ECEF2LLA/Calcul de la latitude/Calcul de mu ==
  xyz_ECEF : Inport
  r : Inport  Port=2
  Constant : Constant
  Product1 : Product
  Selector : Selector  InputPortWidth=3  IndexOptions=Index vector (dialog)  Indices=[3]  OutputSizes=1
  Subtract : Sum  Inputs=+-
  Trigonometric Function : Trigonometry  Operator=atan2
  f : Subsystem
  mu : Outport  VectorParamsAs1DForOutWhenUnconnected=off
  wires:
  Constant/1 -> Subtract/1
  Selector/1 -> Trigonometric Function/1
  f/1(f) -> Subtract/2
  Product1/1 -> Trigonometric Function/2
  r/1 -> Product1/1
  Subtract/1 -> Product1/2
  Trigonometric Function/1 -> mu/1
  xyz_ECEF/1 -> Selector/1

== system MDR_AA_TMD_Intercepteur/Modèle de terre/xyz_NED2LLA/ECEF2LLA/Calcul de la latitude/den(Phi) ==
  mu : Inport
  r : Inport  Port=2
  Constant : Constant  Value=a
  Constant1 : Constant  Value=e
  Constant2 : Constant  Value=3
  Math Function : Math  Operator=magnitude^2  SaturateOnIntegerOverflow=on
  Math Function1 : Math  Operator=pow  SaturateOnIntegerOverflow=on
  Product1 : Product  Inputs=3
  Subtract : Sum  Inputs=+-
  Trigonometric Function : Trigonometry  Operator=cos
  den_phi : Outport  VectorParamsAs1DForOutWhenUnconnected=off
  wires:
  Constant/1 -> Product1/2
  Constant1/1 -> Math Function/1
  mu/1 -> Trigonometric Function/1
  Trigonometric Function/1 -> Math Function1/1
  Constant2/1 -> Math Function1/2
  Math Function/1 -> Product1/3
  Math Function1/1 -> Product1/1
  r/1 -> Subtract/1
  Product1/1 -> Subtract/2
  Subtract/1 -> den_phi/1

== system MDR_AA_TMD_Intercepteur/Modèle de terre/xyz_NED2LLA/ECEF2LLA/Calcul de la latitude/num(Phi) ==
  mu : Inport
  xyz_ECEF : Inport  Port=2
  Add : Sum
  Constant : Constant  Value=b
  Constant1 : Constant  Value=e
  Constant2 : Constant  Value=3
  Math Function : Math  Operator=magnitude^2  SaturateOnIntegerOverflow=on
  Math Function1 : Math  Operator=pow  SaturateOnIntegerOverflow=on
  Product1 : Product  Inputs=3
  Selector : Selector  InputPortWidth=3  IndexOptions=Index vector (dialog)  Indices=[3]  OutputSizes=1
  Trigonometric Function : Trigonometry
  num_phi : Outport  VectorParamsAs1DForOutWhenUnconnected=off
  wires:
  Math Function1/1 -> Product1/1
  Math Function/1 -> Product1/3
  Constant2/1 -> Math Function1/2
  Trigonometric Function/1 -> Math Function1/1
  mu/1 -> Trigonometric Function/1
  Constant1/1 -> Math Function/1
  Constant/1 -> Product1/2
  Product1/1 -> Add/1
  Add/1 -> num_phi/1
  xyz_ECEF/1 -> Selector/1
  Selector/1 -> Add/2

== system MDR_AA_TMD_Intercepteur/Modèle de terre/xyz_NED2LLA/ECEF2LLA/Calcul de r/Norme ==
  V : Inport
  Dot Product : DotProduct  InputSameDT=on  OutDataTypeStr=Inherit: Inherit via internal rule
  Sqrt : Math  Operator=sqrt  SaturateOnIntegerOverflow=on
  ||V|| : Outport  VectorParamsAs1DForOutWhenUnconnected=off
  wires:
  Sqrt/1 -> ||V||/1
  V/1 -> Dot Product/2, Dot Product/1
  Dot Product/1 -> Sqrt/1

== system MDR_AA_TMD_Intercepteur/Modèle de terre/xyz_NED2LLA/xyz_ENU2ECEF/Matrice de passage du repère NED au repère ECEF/Col 1 ==
  Gain : Gain  Gain=-1
  Gain1 : Gain  Gain=-1
  Product : Product
  Product1 : Product
  Trigonometric Function : Trigonometry  Operator=cos
  Trigonometric Function1 : Trigonometry
  Trigonometric Function2 : Trigonometry
  Trigonometric Function3 : Trigonometry
  Trigonometric Function4 : Trigonometry  Operator=cos
  Vector Concatenate : Concatenate  NumInputs=3
  lat0 : Constant  Value=Phi0
  lon0 : Constant  Value=Lambda0
  C1 : Outport  VectorParamsAs1DForOutWhenUnconnected=off
  wires:
  Vector Concatenate/1 -> C1/1
  lat0/1 -> Trigonometric Function4/1, Trigonometric Function2/1, Trigonometric Function1/1
  lon0/1 -> Trigonometric Function3/1, Trigonometric Function/1
  Product/1 -> Gain/1
  Trigonometric Function1/1 -> Product/1
  Trigonometric Function/1 -> Product/2
  Product1/1 -> Gain1/1
  Trigonometric Function3/1 -> Product1/2
  Trigonometric Function2/1 -> Product1/1
  Trigonometric Function4/1 -> Vector Concatenate/3
  Gain/1 -> Vector Concatenate/1
  Gain1/1 -> Vector Concatenate/2

== system MDR_AA_TMD_Intercepteur/Modèle de terre/xyz_NED2LLA/xyz_ENU2ECEF/Matrice de passage du repère NED au repère ECEF/Col 2 ==
  Constant : Constant  Value=0
  Gain2 : Gain  Gain=-1
  Trigonometric Function1 : Trigonometry  Operator=cos
  Trigonometric Function5 : Trigonometry
  Vector Concatenate : Concatenate  NumInputs=3
  lon0 : Constant  Value=Lambda0
  C2 : Outport  VectorParamsAs1DForOutWhenUnconnected=off
  wires:
  Constant/1 -> Vector Concatenate/3
  Trigonometric Function1/1 -> Vector Concatenate/2
  Gain2/1 -> Vector Concatenate/1
  Trigonometric Function5/1 -> Gain2/1
  lon0/1 -> Trigonometric Function1/1, Trigonometric Function5/1
  Vector Concatenate/1 -> C2/1

== system MDR_AA_TMD_Intercepteur/Modèle de terre/xyz_NED2LLA/xyz_ENU2ECEF/Matrice de passage du repère NED au repère ECEF/Col 3 ==
  Gain1 : Gain  Gain=-1
  Gain2 : Gain  Gain=-1
  Gain3 : Gain  Gain=-1
  Product : Product
  Product1 : Product
  Trigonometric Function : Trigonometry  Operator=cos
  Trigonometric Function1 : Trigonometry  Operator=cos
  Trigonometric Function2 : Trigonometry  Operator=cos
  Trigonometric Function3 : Trigonometry
  Trigonometric Function4 : Trigonometry
  Vector Concatenate : Concatenate  NumInputs=3
  lat0 : Constant  Value=Phi0
  lon0 : Constant  Value=Lambda0
  C3 : Outport  VectorParamsAs1DForOutWhenUnconnected=off
  wires:
  Trigonometric Function2/1 -> Product1/1
  Trigonometric Function3/1 -> Product1/2
  Gain3/1 -> Vector Concatenate/2
  Trigonometric Function/1 -> Product/2
  Trigonometric Function1/1 -> Product/1
  Gain2/1 -> Vector Concatenate/1
  Product/1 -> Gain2/1
  lon0/1 -> Trigonometric Function/1, Trigonometric Function3/1
  lat0/1 -> Trigonometric Function1/1, Trigonometric Function2/1, Trigonometric Function4/1
  Product1/1 -> Gain3/1
  Vector Concatenate/1 -> C3/1
  Trigonometric Function4/1 -> Gain1/1
  Gain1/1 -> Vector Concatenate/3

== system MDR_AA_TMD_Intercepteur/Modèle de terre/xyz_NED2LLA/xyz_ENU2ECEF/XYZ0/(1-e^2) ==
  Constant : Constant
  Math Function : Math  Operator=magnitude^2  SaturateOnIntegerOverflow=on
  Sum : Sum  Inputs=|+-
  e : Constant  Value=e
  (1-e^2) : Outport  VectorParamsAs1DForOutWhenUnconnected=off
  wires:
  e/1 -> Math Function/1
  Sum/1 -> (1-e^2)/1
  Math Function/1 -> Sum/2
  Constant/1 -> Sum/1

== system MDR_AA_TMD_Intercepteur/Modèle de terre/xyz_NED2LLA/xyz_ENU2ECEF/XYZ0/Calcul du rayon local ==
  1 : Constant
  Divide : Product  Inputs=*/
  Math Function : Math  Operator=magnitude^2  SaturateOnIntegerOverflow=on
  Math Function1 : Math  Operator=magnitude^2  SaturateOnIntegerOverflow=on
  Product : Product
  Sqrt : Sqrt  SaturateOnIntegerOverflow=on
  Subtract : Sum  Inputs=+-
  Trigonometric Function : Trigonometry
  a : Constant  Value=a
  e : Constant  Value=e
  lat0 : Constant  Value=Phi0
  localradius : Outport  VectorParamsAs1DForOutWhenUnconnected=off
  wires:
  lat0/1 -> Trigonometric Function/1
  Math Function/1 -> Product/1
  a/1 -> Divide/1
  Trigonometric Function/1 -> Math Function1/1
  Sqrt/1 -> Divide/2
  Divide/1 -> localradius/1
  Math Function1/1 -> Product/2
  1/1 -> Subtract/1
  e/1 -> Math Function/1
  Subtract/1 -> Sqrt/1
  Product/1 -> Subtract/2

== system MDR_AA_TMD_Intercepteur/Cible/Cible Cinématique v1.1/Cinématique 6ddl Simulight avec pilotage en force/Calcul des pqr/pqr_a/dérive alpha//beta ==
  AlphaR : Inport
  BetaR : Inport  Port=2
  Clock : Clock
  Divide : Product  Inputs=*/
  Divide1 : Product  Inputs=*/
  IC : InitialCondition
  Memory : Memory
  Memory1 : Memory
  Memory2 : Memory
  Sum : Sum  Inputs=|+-
  Sum1 : Sum  Inputs=|+-
  Sum2 : Sum  Inputs=|+-
  dAlphaR : Outport  VectorParamsAs1DForOutWhenUnconnected=off
  dBetaR : Outport  Port=2  VectorParamsAs1DForOutWhenUnconnected=off
  wires:
  AlphaR/1 -> Memory/1, Sum/1
  Memory/1 -> Sum/2
  Sum/1 -> Divide/1
  BetaR/1 -> Sum1/1, Memory1/1
  Memory1/1 -> Sum1/2
  Sum1/1 -> Divide1/1
  Divide/1 -> dAlphaR/1
  Divide1/1 -> dBetaR/1
  Clock/1 -> Memory2/1, Sum2/1
  Memory2/1 -> Sum2/2
  Sum2/1 -> IC/1
  IC/1 -> Divide1/2, Divide/2

== system MDR_AA_TMD_Intercepteur/Cible/Cible Cinématique v1.1/Cinématique 6ddl Simulight avec pilotage en force/Equations des forces/Gestion de sortie de rampe/Norme ==
  V : Inport
  Dot Product : DotProduct  InputSameDT=on  OutDataTypeStr=Inherit: Inherit via internal rule
  Sqrt : Math  Operator=sqrt  SaturateOnIntegerOverflow=on
  ||V|| : Outport  VectorParamsAs1DForOutWhenUnconnected=off
  wires:
  Sqrt/1 -> ||V||/1
  V/1 -> Dot Product/2, Dot Product/1
  Dot Product/1 -> Sqrt/1
